simulink model "position_velocity_current_control"  (R2024b)
settings: Solver=VariableStepAuto  StartTime=0.0  StopTime=50  FixedStep=1e-5  RelTol=1e-3
values from neighbouring files (symbols this model uses):
  enable_saturators = true    [tuning.m]
  sinusoidal_trajectory = matlabFunction(sinusoidal_trajectory,Vars=[t, f, A])    [trajectories.m]
undefined symbols (not defined in the file or in its folder): b, J, K, Kv, V_nominal
libraries: fl_lib x22, cstblocks x16, nesl_utility x12, ee_lib x2
settings Model: Creator=frenci  LastModifiedBy=enrico
settings RTWCC: GPUComputeCapability=3.5

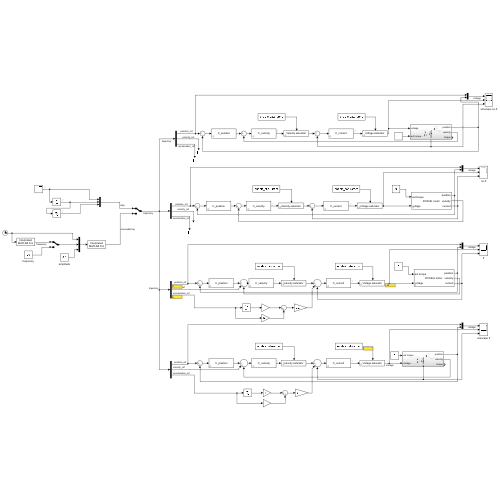
[thumbnail: Simulink's stored preview of the top-level diagram]
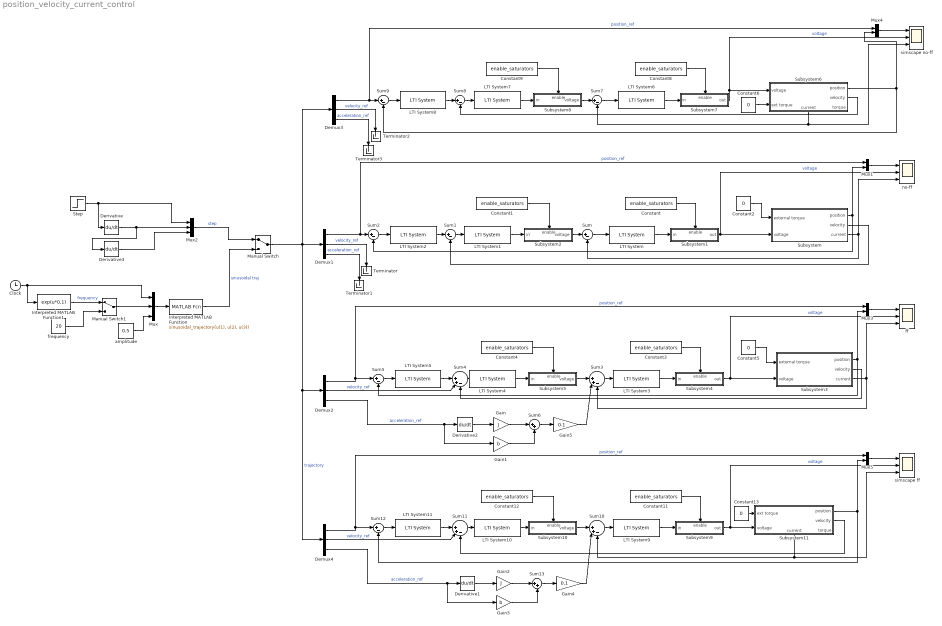
== system position_velocity_current_control ==
  Clock : Clock
  Constant{,1,3..4,8..9,11..12} (8 alike) : Constant  Value=enable_saturators
  Constant{2,5..6,13} (4 alike) : Constant  Value=0
  Demux{1..4} (4 alike) : Demux  Outputs=3
  Derivative : Derivative  CoefficientInTFapproximation=1000
  Derivative1 : Derivative
  Derivative2 : Derivative
  Derivative3 : Derivative  CoefficientInTFapproximation=1000
  Gain : Gain  Gain=J
  Gain1 : Gain  Gain=b
  Gain2 : Gain  Gain=J
  Gain3 : Gain  Gain=b
  Gain4 : Gain  Gain=0.1
  Gain5 : Gain  Gain=0.1
  Interpreted MATLAB Function : MATLABFcn  MATLABFcn=sinusoidal_trajectory(u(1), u(2), u(3))
  Interpreted MATLAB Function1 : MATLABFcn  MATLABFcn=exp(u*0.1)
  LTI System{,3,6,9} (4 alike) : cstblocks/LTI System  sys=C_current  IC=[]  PadeOrder=0
  LTI System{1,4,7,10} (4 alike) : cstblocks/LTI System  sys=C_velocity  IC=[]  PadeOrder=0
  LTI System{2,5,8,11} (4 alike) : cstblocks/LTI System  sys=C_position  IC=[]  PadeOrder=0
  Manual Switch : ManualSwitch
  Manual Switch1 : ManualSwitch
  Mux : Mux  Inputs=3
  Mux{1,3..5} (4 alike) : Mux  Inputs=2
  Mux2 : Mux  Inputs=3
  Step : Step  Time=0.5  SampleTime=0
  Subsystem : Subsystem
      mask Display:
      | disp('DCX22L motor');
      | 
      | port_label('output', 1, 'position');
      | port_label('output', 2, 'velocity');
      | port_label('output', 3, 'current');
      | 
      | port_label('input', 1, 'ext torque');
      | port_label('input', 2, 'voltage');
  Subsystem1 : Subsystem
      settings: PortSchema="{\"entries\":[{\"content\":{\"sides\":[{\"content\":{\"connectorIds\":[\"In1\"]},\"type\":\"ConnectorPlacement.EquallySpacedRectSide\",\"uuid\":\"5670bc23-5208-4592-a101-65e5ca02f12e\"},{\"content\":{\"connectorIds\":[\"Out1\"],\"side\":\"RIGHT\"},\"type\":\"ConnectorPlacement.EquallySpacedRectSide\",\"uuid\":\"ade26b55-5ce8-40ce-8bb9-a19330a12934\"},{\"content\":{\"connectorIds\":[\"In2\"],\"side\":\"TOP\"},\"type\":\"ConnectorPlacement.EquallySpacedRectSide\",\"uuid\":\"b961c51e-f004-41f7-8ef2-708d4a781ba3\"}]},\"type\":\"ConnectorPlacement.EquallySpacedConnector\",\"uuid\":\"606723ef-bc2b-476a-806f-27cbba92a2c4\"}],\"packageUris\":[\"http://schema.mathworks.com/mf0/Connector/R2020b\"],\"version\":\"1.0\"}"
      mask Display: disp('Voltage saturator')
  Subsystem10 : Subsystem
      settings: PortSchema="{\"entries\":[{\"content\":{\"sides\":[{\"content\":{\"connectorIds\":[\"In1\"]},\"type\":\"ConnectorPlacement.EquallySpacedRectSide\",\"uuid\":\"5670bc23-5208-4592-a101-65e5ca02f12e\"},{\"content\":{\"connectorIds\":[\"Out1\"],\"side\":\"RIGHT\"},\"type\":\"ConnectorPlacement.EquallySpacedRectSide\",\"uuid\":\"ade26b55-5ce8-40ce-8bb9-a19330a12934\"},{\"content\":{\"connectorIds\":[\"In2\"],\"side\":\"TOP\"},\"type\":\"ConnectorPlacement.EquallySpacedRectSide\",\"uuid\":\"b961c51e-f004-41f7-8ef2-708d4a781ba3\"}]},\"type\":\"ConnectorPlacement.EquallySpacedConnector\",\"uuid\":\"606723ef-bc2b-476a-806f-27cbba92a2c4\"}],\"packageUris\":[\"http://schema.mathworks.com/mf0/Connector/R2020b\"],\"version\":\"1.0\"}"
      mask Display: disp('Velocity saturator')
  Subsystem11 : Subsystem
      settings: PortSchema="{\"entries\":[{\"content\":{\"sides\":[{\"content\":{\"connectorIds\":[\"In1\",\"In2\"]},\"type\":\"ConnectorPlacement.EquallySpacedRectSide\",\"uuid\":\"c67ff89c-931e-4bc2-864c-883be475405e\"},{\"content\":{\"connectorIds\":[\"Out1\",\"Out2\",\"Out3\"],\"side\":\"RIGHT\"},\"type\":\"ConnectorPlacement.EquallySpacedRectSide\",\"uuid\":\"fb005381-2940-49c3-8bd1-e171080baf17\"},{\"content\":{\"side\":\"TOP\"},\"type\":\"ConnectorPlacement.EquallySpacedRectSide\",\"uuid\":\"7776594d-d5e0-4f5d-a5af-57046ad01644\"},{\"content\":{\"connectorIds\":[\"Out4\"],\"side\":\"BOTTOM\"},\"type\":\"ConnectorPlacement.EquallySpacedRectSide\",\"uuid\":\"24f18840-e2d9-4fce-8caf-60e308a91e4e\"}]},\"type\":\"ConnectorPlacement.EquallySpacedConnector\",\"uuid\":\"98be6553-19ec-40f8-9ca9-83476df98897\"}],\"packageUris\":[\"http://schema.mathworks.com/mf0/Connector/R2020b\"],\"version\":\"1.0\"}"
  Subsystem2 : Subsystem
      settings: PortSchema="{\"entries\":[{\"content\":{\"sides\":[{\"content\":{\"connectorIds\":[\"In1\"]},\"type\":\"ConnectorPlacement.EquallySpacedRectSide\",\"uuid\":\"5670bc23-5208-4592-a101-65e5ca02f12e\"},{\"content\":{\"connectorIds\":[\"Out1\"],\"side\":\"RIGHT\"},\"type\":\"ConnectorPlacement.EquallySpacedRectSide\",\"uuid\":\"ade26b55-5ce8-40ce-8bb9-a19330a12934\"},{\"content\":{\"connectorIds\":[\"In2\"],\"side\":\"TOP\"},\"type\":\"ConnectorPlacement.EquallySpacedRectSide\",\"uuid\":\"b961c51e-f004-41f7-8ef2-708d4a781ba3\"}]},\"type\":\"ConnectorPlacement.EquallySpacedConnector\",\"uuid\":\"606723ef-bc2b-476a-806f-27cbba92a2c4\"}],\"packageUris\":[\"http://schema.mathworks.com/mf0/Connector/R2020b\"],\"version\":\"1.0\"}"
      mask Display: disp('Velocity saturator')
  Subsystem3 : Subsystem
      mask Display:
      | disp('DCX22L motor');
      | 
      | port_label('output', 1, 'position');
      | port_label('output', 2, 'velocity');
      | port_label('output', 3, 'current');
      | 
      | port_label('input', 1, 'ext torque');
      | port_label('input', 2, 'voltage');
  Subsystem4 : Subsystem
      settings: PortSchema="{\"entries\":[{\"content\":{\"sides\":[{\"content\":{\"connectorIds\":[\"In1\"]},\"type\":\"ConnectorPlacement.EquallySpacedRectSide\",\"uuid\":\"5670bc23-5208-4592-a101-65e5ca02f12e\"},{\"content\":{\"connectorIds\":[\"Out1\"],\"side\":\"RIGHT\"},\"type\":\"ConnectorPlacement.EquallySpacedRectSide\",\"uuid\":\"ade26b55-5ce8-40ce-8bb9-a19330a12934\"},{\"content\":{\"connectorIds\":[\"In2\"],\"side\":\"TOP\"},\"type\":\"ConnectorPlacement.EquallySpacedRectSide\",\"uuid\":\"b961c51e-f004-41f7-8ef2-708d4a781ba3\"}]},\"type\":\"ConnectorPlacement.EquallySpacedConnector\",\"uuid\":\"606723ef-bc2b-476a-806f-27cbba92a2c4\"}],\"packageUris\":[\"http://schema.mathworks.com/mf0/Connector/R2020b\"],\"version\":\"1.0\"}"
      mask Display: disp('Voltage saturator')
  Subsystem5 : Subsystem
      settings: PortSchema="{\"entries\":[{\"content\":{\"sides\":[{\"content\":{\"connectorIds\":[\"In1\"]},\"type\":\"ConnectorPlacement.EquallySpacedRectSide\",\"uuid\":\"5670bc23-5208-4592-a101-65e5ca02f12e\"},{\"content\":{\"connectorIds\":[\"Out1\"],\"side\":\"RIGHT\"},\"type\":\"ConnectorPlacement.EquallySpacedRectSide\",\"uuid\":\"ade26b55-5ce8-40ce-8bb9-a19330a12934\"},{\"content\":{\"connectorIds\":[\"In2\"],\"side\":\"TOP\"},\"type\":\"ConnectorPlacement.EquallySpacedRectSide\",\"uuid\":\"b961c51e-f004-41f7-8ef2-708d4a781ba3\"}]},\"type\":\"ConnectorPlacement.EquallySpacedConnector\",\"uuid\":\"606723ef-bc2b-476a-806f-27cbba92a2c4\"}],\"packageUris\":[\"http://schema.mathworks.com/mf0/Connector/R2020b\"],\"version\":\"1.0\"}"
      mask Display: disp('Velocity saturator')
  Subsystem6 : Subsystem
      settings: PortSchema="{\"entries\":[{\"content\":{\"sides\":[{\"content\":{\"connectorIds\":[\"In1\",\"In2\"]},\"type\":\"ConnectorPlacement.EquallySpacedRectSide\",\"uuid\":\"c67ff89c-931e-4bc2-864c-883be475405e\"},{\"content\":{\"connectorIds\":[\"Out1\",\"Out2\",\"Out3\"],\"side\":\"RIGHT\"},\"type\":\"ConnectorPlacement.EquallySpacedRectSide\",\"uuid\":\"fb005381-2940-49c3-8bd1-e171080baf17\"},{\"content\":{\"side\":\"TOP\"},\"type\":\"ConnectorPlacement.EquallySpacedRectSide\",\"uuid\":\"7776594d-d5e0-4f5d-a5af-57046ad01644\"},{\"content\":{\"connectorIds\":[\"Out4\"],\"side\":\"BOTTOM\"},\"type\":\"ConnectorPlacement.EquallySpacedRectSide\",\"uuid\":\"24f18840-e2d9-4fce-8caf-60e308a91e4e\"}]},\"type\":\"ConnectorPlacement.EquallySpacedConnector\",\"uuid\":\"98be6553-19ec-40f8-9ca9-83476df98897\"}],\"packageUris\":[\"http://schema.mathworks.com/mf0/Connector/R2020b\"],\"version\":\"1.0\"}"
  Subsystem7 : Subsystem
      settings: PortSchema="{\"entries\":[{\"content\":{\"sides\":[{\"content\":{\"connectorIds\":[\"In1\"]},\"type\":\"ConnectorPlacement.EquallySpacedRectSide\",\"uuid\":\"5670bc23-5208-4592-a101-65e5ca02f12e\"},{\"content\":{\"connectorIds\":[\"Out1\"],\"side\":\"RIGHT\"},\"type\":\"ConnectorPlacement.EquallySpacedRectSide\",\"uuid\":\"ade26b55-5ce8-40ce-8bb9-a19330a12934\"},{\"content\":{\"connectorIds\":[\"In2\"],\"side\":\"TOP\"},\"type\":\"ConnectorPlacement.EquallySpacedRectSide\",\"uuid\":\"b961c51e-f004-41f7-8ef2-708d4a781ba3\"}]},\"type\":\"ConnectorPlacement.EquallySpacedConnector\",\"uuid\":\"606723ef-bc2b-476a-806f-27cbba92a2c4\"}],\"packageUris\":[\"http://schema.mathworks.com/mf0/Connector/R2020b\"],\"version\":\"1.0\"}"
      mask Display: disp('Voltage saturator')
  Subsystem8 : Subsystem
      settings: PortSchema="{\"entries\":[{\"content\":{\"sides\":[{\"content\":{\"connectorIds\":[\"In1\"]},\"type\":\"ConnectorPlacement.EquallySpacedRectSide\",\"uuid\":\"5670bc23-5208-4592-a101-65e5ca02f12e\"},{\"content\":{\"connectorIds\":[\"Out1\"],\"side\":\"RIGHT\"},\"type\":\"ConnectorPlacement.EquallySpacedRectSide\",\"uuid\":\"ade26b55-5ce8-40ce-8bb9-a19330a12934\"},{\"content\":{\"connectorIds\":[\"In2\"],\"side\":\"TOP\"},\"type\":\"ConnectorPlacement.EquallySpacedRectSide\",\"uuid\":\"b961c51e-f004-41f7-8ef2-708d4a781ba3\"}]},\"type\":\"ConnectorPlacement.EquallySpacedConnector\",\"uuid\":\"606723ef-bc2b-476a-806f-27cbba92a2c4\"}],\"packageUris\":[\"http://schema.mathworks.com/mf0/Connector/R2020b\"],\"version\":\"1.0\"}"
      mask Display: disp('Velocity saturator')
  Subsystem9 : Subsystem
      settings: PortSchema="{\"entries\":[{\"content\":{\"sides\":[{\"content\":{\"connectorIds\":[\"In1\"]},\"type\":\"ConnectorPlacement.EquallySpacedRectSide\",\"uuid\":\"5670bc23-5208-4592-a101-65e5ca02f12e\"},{\"content\":{\"connectorIds\":[\"Out1\"],\"side\":\"RIGHT\"},\"type\":\"ConnectorPlacement.EquallySpacedRectSide\",\"uuid\":\"ade26b55-5ce8-40ce-8bb9-a19330a12934\"},{\"content\":{\"connectorIds\":[\"In2\"],\"side\":\"TOP\"},\"type\":\"ConnectorPlacement.EquallySpacedRectSide\",\"uuid\":\"b961c51e-f004-41f7-8ef2-708d4a781ba3\"}]},\"type\":\"ConnectorPlacement.EquallySpacedConnector\",\"uuid\":\"606723ef-bc2b-476a-806f-27cbba92a2c4\"}],\"packageUris\":[\"http://schema.mathworks.com/mf0/Connector/R2020b\"],\"version\":\"1.0\"}"
      mask Display: disp('Voltage saturator')
  Sum{,1..2,5,7..9,12} (8 alike) : Sum  Inputs=|+-
  Sum{3..4,10..11} (4 alike) : Sum  Inputs=||++-
  Sum13 : Sum  Inputs=|++
  Sum6 : Sum  Inputs=|++
  Terminator{,1..3} (4 alike) : Terminator
  amplitude : Constant  Value=0.5
  ff : Scope  NumInputPorts=3
  frequency : Constant  Value=20
  no-ff : Scope  NumInputPorts=3
  simscape ff : Scope  NumInputPorts=3
  simscape no-ff : Scope  NumInputPorts=3
  wires:
  LTI System/1 -> Subsystem1/1(in)
  Subsystem1/1(out) -> no-ff/2, Subsystem/2(voltage)  "voltage"
  Sum/1 -> LTI System/1
  Subsystem/3(current) -> Sum/2, no-ff/3
  Sum1/1 -> LTI System1/1
  LTI System1/1 -> Subsystem2/1(in)
  Subsystem2/1(voltage) -> Sum/1
  LTI System2/1 -> Sum1/1
  Subsystem/2(velocity) -> Sum1/2
  Subsystem/1(position) -> Mux1/2, Sum2/2
  Sum2/1 -> LTI System2/1
  Demux1/1 -> Mux1/1, Sum2/1  "position_ref"
  Mux/1 -> Interpreted MATLAB Function/1
  Clock/1 -> Interpreted MATLAB Function1/1, Mux/1
  Manual Switch1/1 -> Mux/2
  Interpreted MATLAB Function/1 -> Manual Switch/2  "sinusoidal traj"
  amplitude/1 -> Mux/3
  Constant2/1 -> Subsystem/1(external torque)
  Constant/1 -> Subsystem1/2(enable)
  Constant1/1 -> Subsystem2/2(enable)
  Mux1/1 -> no-ff/1
  Step/1 -> Derivative/1, Mux2/1
  Mux2/1 -> Manual Switch/1  "step"
  Constant4/1 -> Subsystem5/2(enable)
  Constant5/1 -> Subsystem3/1(external torque)
  Subsystem3/3(current) -> ff/3, Sum3/3
  Constant3/1 -> Subsystem4/2(enable)
  Subsystem5/1(voltage) -> Sum3/1
  LTI System5/1 -> Sum4/1
  Demux2/1 -> Mux3/1, Sum5/1  "position_ref"
  Subsystem4/1(out) -> ff/2, Subsystem3/2(voltage)  "voltage"
  Subsystem3/1(position) -> Mux3/2, Sum5/2
  LTI System4/1 -> Subsystem5/1(in)
  LTI System3/1 -> Subsystem4/1(in)
  Sum3/1 -> LTI System3/1
  Sum4/1 -> LTI System4/1
  Subsystem3/2(velocity) -> Sum4/3
  Sum5/1 -> LTI System5/1
  Demux2/2 -> Sum4/2  "velocity_ref"
  Demux2/3 -> Derivative2/1, Gain1/1  "acceleration_ref"
  Derivative2/1 -> Gain/1
  Gain1/1 -> Sum6/2
  Gain/1 -> Sum6/1
  Sum6/1 -> Gain5/1
  Demux1/2 -> Terminator/1  "velocity_ref"
  Mux3/1 -> ff/1
  Demux1/3 -> Terminator1/1  "acceleration_ref"
  Subsystem6/4(current) -> simscape no-ff/3, Sum7/2
  Constant8/1 -> Subsystem7/2(enable)
  LTI System8/1 -> Sum8/1
  Mux4/1 -> simscape no-ff/1
  Subsystem8/1(voltage) -> Sum7/1
  Demux3/1 -> Mux4/1, Sum9/1  "position_ref"
  Demux3/2 -> Terminator2/1  "velocity_ref"
  Sum8/1 -> LTI System7/1
  Subsystem7/1(out) -> simscape no-ff/2, Subsystem6/1(voltage)  "voltage"
  Demux3/3 -> Terminator3/1  "acceleration_ref"
  LTI System6/1 -> Subsystem7/1(in)
  Constant9/1 -> Subsystem8/2(enable)
  LTI System7/1 -> Subsystem8/1(in)
  Sum7/1 -> LTI System6/1
  Sum9/1 -> LTI System8/1
  LTI System11/1 -> Sum11/1
  Constant12/1 -> Subsystem10/2(enable)
  Constant11/1 -> Subsystem9/2(enable)
  Sum12/1 -> LTI System11/1
  Subsystem11/2(velocity) -> Sum11/3
  Sum10/1 -> LTI System9/1
  LTI System9/1 -> Subsystem9/1(in)
  LTI System10/1 -> Subsystem10/1(in)
  Gain2/1 -> Sum13/1
  Subsystem9/1(out) -> Subsystem11/2(voltage), simscape ff/2  "voltage"
  Demux4/1 -> Mux5/1, Sum12/1  "position_ref"
  Subsystem10/1(voltage) -> Sum10/1
  Sum11/1 -> LTI System10/1
  Derivative1/1 -> Gain2/1
  Sum13/1 -> Gain4/1
  Mux5/1 -> simscape ff/1
  Demux4/2 -> Sum11/2  "velocity_ref"
  Subsystem11/1(position) -> Sum12/2, Mux5/2
  Gain3/1 -> Sum13/2
  Manual Switch/1 -> Demux3/1, Demux4/1, Demux2/1, Demux1/1  "trajectory"
  Subsystem11/4(current) -> simscape ff/3, Sum10/3
  Demux4/3 -> Derivative1/1, Gain3/1  "acceleration_ref"
  Derivative/1 -> Derivative3/1, Mux2/2
  Derivative3/1 -> Mux2/3
  Subsystem6/2(velocity) -> Sum8/2
  Subsystem6/1(position) -> Sum9/2, Mux4/2
  Constant6/1 -> Subsystem6/2(ext torque)
  Constant13/1 -> Subsystem11/1(ext torque)
  Gain4/1 -> Sum10/2
  Interpreted MATLAB Function1/1 -> Manual Switch1/1  "frequency"
  frequency/1 -> Manual Switch1/2
  Gain5/1 -> Sum3/2

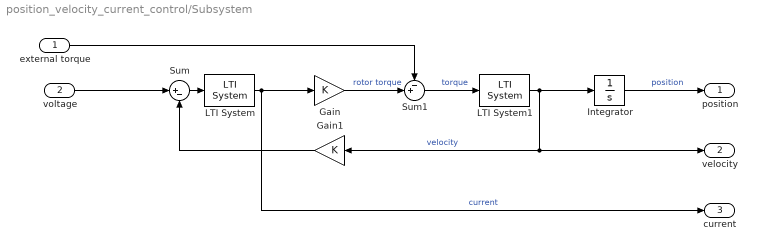
== system position_velocity_current_control/Subsystem ==
  external torque : Inport
  voltage : Inport  Port=2
  Gain : Gain  Gain=K
  Gain1 : Gain  Gain=K
  Integrator : Integrator
  LTI System : cstblocks/LTI System  sys=El  IC=[]  PadeOrder=0
  LTI System1 : cstblocks/LTI System  sys=Me  IC=[]  PadeOrder=0
  Sum : Sum  Inputs=|+-
  Sum1 : Sum  Inputs=-+|
  position : Outport
  velocity : Outport  Port=2
  current : Outport  Port=3
  wires:
  LTI System/1 -> current/1, Gain/1  "current"
  Gain1/1 -> Sum/2
  Integrator/1 -> position/1  "position"
  voltage/1 -> Sum/1
  Gain/1 -> Sum1/2  "rotor torque"
  Sum1/1 -> LTI System1/1  "torque"
  Sum/1 -> LTI System/1
  LTI System1/1 -> velocity/1, Gain1/1, Integrator/1  "velocity"
  external torque/1 -> Sum1/1

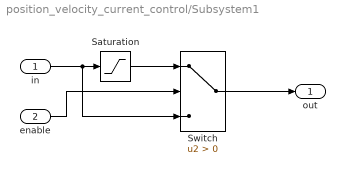
== system position_velocity_current_control/Subsystem1 ==
  in : Inport
  enable : Inport  Port=2
  Saturation : Saturate  UpperLimit=V_nominal  LowerLimit=-V_nominal
  Switch : Switch  Criteria=u2 > Threshold  SaturateOnIntegerOverflow=off  InputSameDT=off
  out : Outport
  wires:
  in/1 -> Switch/3, Saturation/1
  enable/1 -> Switch/2
  Switch/1 -> out/1
  Saturation/1 -> Switch/1

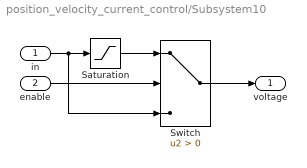
== system position_velocity_current_control/Subsystem10 ==
  in : Inport
  enable : Inport  Port=2
  Saturation : Saturate  UpperLimit=V_nominal*Kv*0.10472  LowerLimit=-V_nominal*Kv*0.10472
  Switch : Switch  Criteria=u2 > Threshold  SaturateOnIntegerOverflow=off  InputSameDT=off
  voltage : Outport
  wires:
  in/1 -> Switch/3, Saturation/1
  Switch/1 -> voltage/1
  Saturation/1 -> Switch/1
  enable/1 -> Switch/2

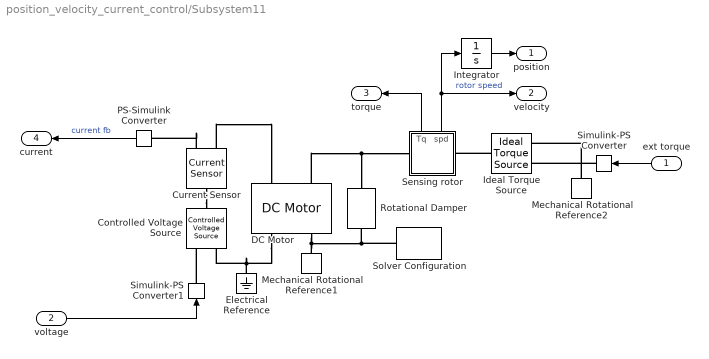
== system position_velocity_current_control/Subsystem11 ==
  ext torque : Inport
  voltage : Inport  Port=2
  Controlled Voltage Source : fl_lib/Electrical/Electrical Sources/Controlled Voltage Source
  Current Sensor : fl_lib/Electrical/Electrical Sensors/Current Sensor
  DC Motor : ee_lib/Electromechanical/Brushed Motors/DC Motor  field_option=ee.enum.field_option.pm  Rf=100 Ohm  Lf=1 H  Laf=0.15 H  If0=0 A  parameterization=ee.enum.dcparam_option.circuit_param  Ra=R Ohm  La=L H  emf_or_torque=ee.enum.emf_or_torque.kv  Kv=1/Kv V/rpm  Ki=6.876e-4 N*m/A  T_stall=0.24e-3 N*m  w_max=19100 rpm  w_rated=15000 rpm  P_rated=0.08 W  V_rated=1.5 V  lam_param=ee.enum.lam_param.current  i_noload="54.6  mA"  V_i_noload=18 V  J=J cm^2*g  lam=0 N*m*s/rad  speed0=0 rpm  t_fault_armature=1 s  t_fault_field=1 s  fault_action=simscape.enum.assert.action.none  alpha=3.93e-3 1/K  Tmeas=25 degC  thermal_mass=100 J/K  initial_temperature=25 degC
  Electrical Reference : fl_lib/Electrical/Electrical Elements/Electrical Reference
  Ideal Torque Source : fl_lib/Mechanical/Mechanical Sources/Ideal Torque Source
  Integrator : Integrator
  Mechanical Rotational Reference1 : fl_lib/Mechanical/Rotational Elements/Mechanical Rotational Reference
  Mechanical Rotational Reference2 : fl_lib/Mechanical/Rotational Elements/Mechanical Rotational Reference
  PS-Simulink Converter : nesl_utility/PS-Simulink Converter  PhysicalDomain=network_engine_domain  SubClassName=ps_output  LeftPortType=input  RightPortType=output  PseudoPeriodic=off  Frequencies=[]  VectorFormat=inherit  Unit=inherit  AffineConversion=off
  Rotational Damper : fl_lib/Mechanical/Rotational Elements/Rotational Damper  D=b N*m*s/rad  w_specify=off  w_priority=None  w=0 rad/s  w_nominal_specify=off  w_nominal_value=1  w_nominal_unit=rad/s  t_specify=off  t_priority=None  t=0 N*m  t_nominal_specify=off  t_nominal_value=1  t_nominal_unit=N*m
  Sensing rotor : Subsystem
      settings: PortSchema="{\"entries\":[{\"content\":{\"sides\":[{\"content\":{\"connectorIds\":[\"LConn1\"]},\"type\":\"ConnectorPlacement.EquallySpacedRectSide\",\"uuid\":\"9165a8ad-3db0-41c0-ab54-3b61ce0d4991\"},{\"content\":{\"connectorIds\":[\"RConn1\"],\"side\":\"RIGHT\"},\"type\":\"ConnectorPlacement.EquallySpacedRectSide\",\"uuid\":\"77dd0fe0-a538-4e9a-a5e5-b4e8faf0921d\"},{\"content\":{\"connectorIds\":[\"Out1\",\"Out2\"],\"side\":\"TOP\"},\"type\":\"ConnectorPlacement.EquallySpacedRectSide\",\"uuid\":\"6454db15-9e49-4f4a-bb19-0d462346e2ce\"},{\"content\":{\"connectorIds\":[],\"side\":\"BOTTOM\"},\"type\":\"ConnectorPlacement.EquallySpacedRectSide\",\"uuid\":\"205718cf-2aa2-41bb-bfb4-a63575d19392\"}]},\"type\":\"ConnectorPlacement.EquallySpacedConnector\",\"uuid\":\"b0e56a53-c948-4e6a-adfb-62f2ad9887fa\"}],\"packageUris\":[\"http://schema.mathworks.com/mf0/Connector/R2020b\"],\"version\":\"1.0\"}"
  Simulink-PS Converter : nesl_utility/Simulink-PS Converter  PhysicalDomain=network_engine_domain  SubClassName=ps_input  LeftPortType=input  RightPortType=output  PseudoPeriodic=off  Frequencies=[]  NoiseDistribution=none  NoiseParameters=[]  Unit=1  AffineConversion=off  FilteringAndDerivatives=provide  SimscapeFilterOrder=1  InputFilterTimeConstant=0.001  UdotUserProvided=0
  Simulink-PS Converter1 : nesl_utility/Simulink-PS Converter  PhysicalDomain=network_engine_domain  SubClassName=ps_input  LeftPortType=input  RightPortType=output  PseudoPeriodic=off  Frequencies=[]  NoiseDistribution=none  NoiseParameters=[]  Unit=1  AffineConversion=off  FilteringAndDerivatives=zero  SimscapeFilterOrder=1  InputFilterTimeConstant=0.001  UdotUserProvided=0
  Solver Configuration : nesl_utility/Solver Configuration  PhysicalDomain=network_engine_domain  SubClassName=solver  LeftPortType=input  RightPortType=generic  Tones=[]  Harmonics=[]  SimulateNoise=off  Profile=off  UseLocalSampling=off  EnableSwitchedLinearOptims=on  FrequencyDomain=off  UseCCode=off  RelTol=0.001  AbsTol=0.001  MinStep=1e-09  ToWorkspace=off  RevertToSquareIcSolve=off  NumHomotopyIterations=100  PhasorMode=off  PhasorModeNumHarmonics=1  ConsistencySolver=NEWTON_XTOL_AFTER_FTOL  IndexReductionMethod=DerivativeReplacement  DoDC=off  ResidualTolerance=1e-09  ConsistencyTolSource=GLOBAL  ConsistencyAbsTol=0.001  ConsistencyRelTol=0.001  ConsistencyTolFactor=0.000001  UseLocalSolver=off  LocalSolverChoice=NE_BACKWARD_EULER_ADVANCER  ResolveIndetEquations=on  FunctionEvalNumThread=1  LocalSolverSampleTime=0.001  DoFixedCost=off  MaxNonlinIter=3  MaxModeIter=2  ComputeImpulses=off  ImpulseIterations=2  LinearAlgebra=auto  LinearAlgebraNumThread=0  EquationFormulation=NE_TIME_EF  DelaysMemoryBudget=1024  AutomaticFiltering=on  FilteringTimeConstant=0.001  PartitionStorageMethod=AS_NEEDED  PartitionMemoryBudget=1024  PartitionMethod=ROBUST  MultibodyUseLocalSolver=off  MultibodyLocalSolverChoice=ODE1  MultibodyLocalSolverSampleTime=0.001
  position : Outport
  velocity : Outport  Port=2
  torque : Outport  Port=3
  current : Outport  Port=4
  wires:
  Sensing rotor/1(Tq) -> torque/1
  PS-Simulink Converter/1 -> current/1  "current fb"
  Sensing rotor/2(spd) -> Integrator/1, velocity/1  "rotor speed"
  voltage/1 -> Simulink-PS Converter1/1
  ext torque/1 -> Simulink-PS Converter/1
  Integrator/1 -> position/1
  connections:
  DC Motor/RConn1 -- Electrical Reference/LConn1 -- Controlled Voltage Source/RConn2
  Current Sensor/RConn1 -- PS-Simulink Converter/LConn1
  Simulink-PS Converter1/RConn1 -- Controlled Voltage Source/RConn1
  DC Motor/LConn2 -- Rotational Damper/LConn1 -- Sensing rotor/LConn1
  DC Motor/RConn2 -- Mechanical Rotational Reference1/LConn1 -- Solver Configuration/RConn1 -- Rotational Damper/RConn1
  Current Sensor/RConn2 -- DC Motor/LConn1
  Ideal Torque Source/LConn1 -- Sensing rotor/RConn1
  Current Sensor/LConn1 -- Controlled Voltage Source/LConn1
  Simulink-PS Converter/RConn1 -- Ideal Torque Source/RConn1
  Mechanical Rotational Reference2/LConn1 -- Ideal Torque Source/RConn2

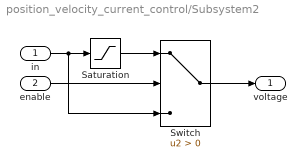
== system position_velocity_current_control/Subsystem2 ==
  in : Inport
  enable : Inport  Port=2
  Saturation : Saturate  UpperLimit=V_nominal*Kv*0.10472  LowerLimit=-V_nominal*Kv*0.10472
  Switch : Switch  Criteria=u2 > Threshold  SaturateOnIntegerOverflow=off  InputSameDT=off
  voltage : Outport
  wires:
  in/1 -> Switch/3, Saturation/1
  Switch/1 -> voltage/1
  Saturation/1 -> Switch/1
  enable/1 -> Switch/2

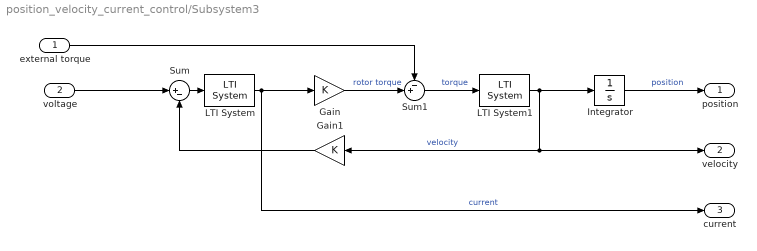
== system position_velocity_current_control/Subsystem3 ==
  external torque : Inport
  voltage : Inport  Port=2
  Gain : Gain  Gain=K
  Gain1 : Gain  Gain=K
  Integrator : Integrator
  LTI System : cstblocks/LTI System  sys=El  IC=[]  PadeOrder=0
  LTI System1 : cstblocks/LTI System  sys=Me  IC=[]  PadeOrder=0
  Sum : Sum  Inputs=|+-
  Sum1 : Sum  Inputs=-+|
  position : Outport
  velocity : Outport  Port=2
  current : Outport  Port=3
  wires:
  LTI System/1 -> current/1, Gain/1  "current"
  Gain1/1 -> Sum/2
  Integrator/1 -> position/1  "position"
  voltage/1 -> Sum/1
  Gain/1 -> Sum1/2  "rotor torque"
  Sum1/1 -> LTI System1/1  "torque"
  Sum/1 -> LTI System/1
  LTI System1/1 -> velocity/1, Gain1/1, Integrator/1  "velocity"
  external torque/1 -> Sum1/1

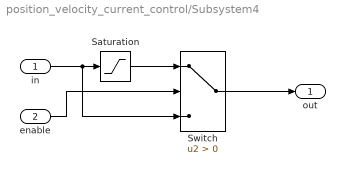
== system position_velocity_current_control/Subsystem4 ==
  in : Inport
  enable : Inport  Port=2
  Saturation : Saturate  UpperLimit=V_nominal  LowerLimit=-V_nominal  ZeroCross=off
  Switch : Switch  Criteria=u2 > Threshold  SaturateOnIntegerOverflow=off  InputSameDT=off
  out : Outport
  wires:
  in/1 -> Switch/3, Saturation/1
  enable/1 -> Switch/2
  Switch/1 -> out/1
  Saturation/1 -> Switch/1

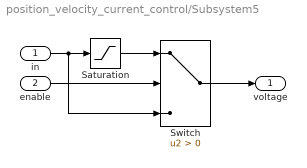
== system position_velocity_current_control/Subsystem5 ==
  in : Inport
  enable : Inport  Port=2
  Saturation : Saturate  UpperLimit=V_nominal*Kv*0.10472  LowerLimit=-V_nominal*Kv*0.10472
  Switch : Switch  Criteria=u2 > Threshold  SaturateOnIntegerOverflow=off  InputSameDT=off
  voltage : Outport
  wires:
  in/1 -> Switch/3, Saturation/1
  Switch/1 -> voltage/1
  Saturation/1 -> Switch/1
  enable/1 -> Switch/2

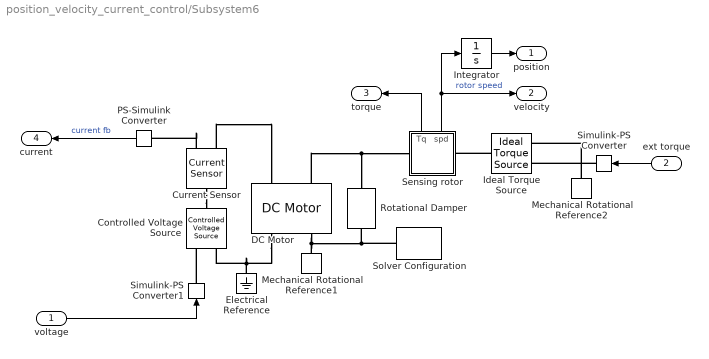
== system position_velocity_current_control/Subsystem6 ==
  voltage : Inport
  ext torque : Inport  Port=2
  Controlled Voltage Source : fl_lib/Electrical/Electrical Sources/Controlled Voltage Source
  Current Sensor : fl_lib/Electrical/Electrical Sensors/Current Sensor
  DC Motor : ee_lib/Electromechanical/Brushed Motors/DC Motor  field_option=ee.enum.field_option.pm  Rf=100 Ohm  Lf=1 H  Laf=0.15 H  If0=0 A  parameterization=ee.enum.dcparam_option.circuit_param  Ra=R Ohm  La=L H  emf_or_torque=ee.enum.emf_or_torque.kv  Kv=1/Kv V/rpm  Ki=6.876e-4 N*m/A  T_stall=0.24e-3 N*m  w_max=19100 rpm  w_rated=15000 rpm  P_rated=0.08 W  V_rated=1.5 V  lam_param=ee.enum.lam_param.current  i_noload="54.6  mA"  V_i_noload=18 V  J=J cm^2*g  lam=0 N*m*s/rad  speed0=0 rpm  t_fault_armature=1 s  t_fault_field=1 s  fault_action=simscape.enum.assert.action.none  alpha=3.93e-3 1/K  Tmeas=25 degC  thermal_mass=100 J/K  initial_temperature=25 degC
  Electrical Reference : fl_lib/Electrical/Electrical Elements/Electrical Reference
  Ideal Torque Source : fl_lib/Mechanical/Mechanical Sources/Ideal Torque Source
  Integrator : Integrator
  Mechanical Rotational Reference1 : fl_lib/Mechanical/Rotational Elements/Mechanical Rotational Reference
  Mechanical Rotational Reference2 : fl_lib/Mechanical/Rotational Elements/Mechanical Rotational Reference
  PS-Simulink Converter : nesl_utility/PS-Simulink Converter  PhysicalDomain=network_engine_domain  SubClassName=ps_output  LeftPortType=input  RightPortType=output  PseudoPeriodic=off  Frequencies=[]  VectorFormat=inherit  Unit=inherit  AffineConversion=off
  Rotational Damper : fl_lib/Mechanical/Rotational Elements/Rotational Damper  D=b N*m*s/rad  w_specify=off  w_priority=None  w=0 rad/s  w_nominal_specify=off  w_nominal_value=1  w_nominal_unit=rad/s  t_specify=off  t_priority=None  t=0 N*m  t_nominal_specify=off  t_nominal_value=1  t_nominal_unit=N*m
  Sensing rotor : Subsystem
      settings: PortSchema="{\"entries\":[{\"content\":{\"sides\":[{\"content\":{\"connectorIds\":[\"LConn1\"]},\"type\":\"ConnectorPlacement.EquallySpacedRectSide\",\"uuid\":\"9165a8ad-3db0-41c0-ab54-3b61ce0d4991\"},{\"content\":{\"connectorIds\":[\"RConn1\"],\"side\":\"RIGHT\"},\"type\":\"ConnectorPlacement.EquallySpacedRectSide\",\"uuid\":\"77dd0fe0-a538-4e9a-a5e5-b4e8faf0921d\"},{\"content\":{\"connectorIds\":[\"Out1\",\"Out2\"],\"side\":\"TOP\"},\"type\":\"ConnectorPlacement.EquallySpacedRectSide\",\"uuid\":\"6454db15-9e49-4f4a-bb19-0d462346e2ce\"},{\"content\":{\"connectorIds\":[],\"side\":\"BOTTOM\"},\"type\":\"ConnectorPlacement.EquallySpacedRectSide\",\"uuid\":\"205718cf-2aa2-41bb-bfb4-a63575d19392\"}]},\"type\":\"ConnectorPlacement.EquallySpacedConnector\",\"uuid\":\"b0e56a53-c948-4e6a-adfb-62f2ad9887fa\"}],\"packageUris\":[\"http://schema.mathworks.com/mf0/Connector/R2020b\"],\"version\":\"1.0\"}"
  Simulink-PS Converter : nesl_utility/Simulink-PS Converter  PhysicalDomain=network_engine_domain  SubClassName=ps_input  LeftPortType=input  RightPortType=output  PseudoPeriodic=off  Frequencies=[]  NoiseDistribution=none  NoiseParameters=[]  Unit=1  AffineConversion=off  FilteringAndDerivatives=provide  SimscapeFilterOrder=1  InputFilterTimeConstant=0.001  UdotUserProvided=0
  Simulink-PS Converter1 : nesl_utility/Simulink-PS Converter  PhysicalDomain=network_engine_domain  SubClassName=ps_input  LeftPortType=input  RightPortType=output  PseudoPeriodic=off  Frequencies=[]  NoiseDistribution=none  NoiseParameters=[]  Unit=1  AffineConversion=off  FilteringAndDerivatives=zero  SimscapeFilterOrder=1  InputFilterTimeConstant=0.001  UdotUserProvided=0
  Solver Configuration : nesl_utility/Solver Configuration  PhysicalDomain=network_engine_domain  SubClassName=solver  LeftPortType=input  RightPortType=generic  Tones=[]  Harmonics=[]  SimulateNoise=off  Profile=off  UseLocalSampling=off  EnableSwitchedLinearOptims=on  FrequencyDomain=off  UseCCode=off  RelTol=0.001  AbsTol=0.001  MinStep=1e-09  ToWorkspace=off  RevertToSquareIcSolve=off  NumHomotopyIterations=100  PhasorMode=off  PhasorModeNumHarmonics=1  ConsistencySolver=NEWTON_XTOL_AFTER_FTOL  IndexReductionMethod=DerivativeReplacement  DoDC=off  ResidualTolerance=1e-09  ConsistencyTolSource=GLOBAL  ConsistencyAbsTol=0.001  ConsistencyRelTol=0.001  ConsistencyTolFactor=0.000001  UseLocalSolver=off  LocalSolverChoice=NE_BACKWARD_EULER_ADVANCER  ResolveIndetEquations=on  FunctionEvalNumThread=1  LocalSolverSampleTime=0.001  DoFixedCost=off  MaxNonlinIter=3  MaxModeIter=2  ComputeImpulses=off  ImpulseIterations=2  LinearAlgebra=auto  LinearAlgebraNumThread=0  EquationFormulation=NE_TIME_EF  DelaysMemoryBudget=1024  AutomaticFiltering=on  FilteringTimeConstant=0.001  PartitionStorageMethod=AS_NEEDED  PartitionMemoryBudget=1024  PartitionMethod=ROBUST  MultibodyUseLocalSolver=off  MultibodyLocalSolverChoice=ODE1  MultibodyLocalSolverSampleTime=0.001
  position : Outport
  velocity : Outport  Port=2
  torque : Outport  Port=3
  current : Outport  Port=4
  wires:
  Sensing rotor/1(Tq) -> torque/1
  PS-Simulink Converter/1 -> current/1  "current fb"
  Sensing rotor/2(spd) -> Integrator/1, velocity/1  "rotor speed"
  voltage/1 -> Simulink-PS Converter1/1
  ext torque/1 -> Simulink-PS Converter/1
  Integrator/1 -> position/1
  connections:
  DC Motor/RConn1 -- Electrical Reference/LConn1 -- Controlled Voltage Source/RConn2
  Current Sensor/RConn1 -- PS-Simulink Converter/LConn1
  Simulink-PS Converter1/RConn1 -- Controlled Voltage Source/RConn1
  DC Motor/LConn2 -- Sensing rotor/LConn1 -- Rotational Damper/LConn1
  DC Motor/RConn2 -- Mechanical Rotational Reference1/LConn1 -- Solver Configuration/RConn1 -- Rotational Damper/RConn1
  Current Sensor/RConn2 -- DC Motor/LConn1
  Ideal Torque Source/LConn1 -- Sensing rotor/RConn1
  Current Sensor/LConn1 -- Controlled Voltage Source/LConn1
  Simulink-PS Converter/RConn1 -- Ideal Torque Source/RConn1
  Mechanical Rotational Reference2/LConn1 -- Ideal Torque Source/RConn2

== system position_velocity_current_control/Subsystem7 ==
  in : Inport
  enable : Inport  Port=2
  Saturation : Saturate  UpperLimit=V_nominal  LowerLimit=-V_nominal
  Switch : Switch  Criteria=u2 > Threshold  SaturateOnIntegerOverflow=off  InputSameDT=off
  out : Outport
  wires:
  in/1 -> Switch/3, Saturation/1
  enable/1 -> Switch/2
  Switch/1 -> out/1
  Saturation/1 -> Switch/1

== system position_velocity_current_control/Subsystem8 ==
  in : Inport
  enable : Inport  Port=2
  Saturation : Saturate  UpperLimit=V_nominal*Kv*0.10472  LowerLimit=-V_nominal*Kv*0.10472
  Switch : Switch  Criteria=u2 > Threshold  SaturateOnIntegerOverflow=off  InputSameDT=off
  voltage : Outport
  wires:
  in/1 -> Switch/3, Saturation/1
  Switch/1 -> voltage/1
  Saturation/1 -> Switch/1
  enable/1 -> Switch/2

== system position_velocity_current_control/Subsystem9 ==
  in : Inport
  enable : Inport  Port=2
  Saturation : Saturate  UpperLimit=V_nominal  LowerLimit=-V_nominal  ZeroCross=off
  Switch : Switch  Criteria=u2 > Threshold  SaturateOnIntegerOverflow=off  InputSameDT=off
  out : Outport
  wires:
  in/1 -> Switch/3, Saturation/1
  enable/1 -> Switch/2
  Switch/1 -> out/1
  Saturation/1 -> Switch/1

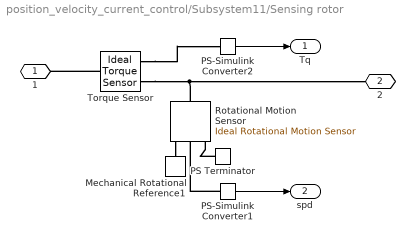
== system position_velocity_current_control/Subsystem11/Sensing rotor ==
  Mechanical Rotational Reference1 : fl_lib/Mechanical/Rotational Elements/Mechanical Rotational Reference
  PS Terminator : fl_lib/Physical Signals/Sinks/PS Terminator
  PS-Simulink Converter1 : nesl_utility/PS-Simulink Converter  PhysicalDomain=network_engine_domain  SubClassName=ps_output  LeftPortType=input  RightPortType=output  PseudoPeriodic=off  Frequencies=[]  VectorFormat=1-D array  Unit=rpm  AffineConversion=off
  PS-Simulink Converter2 : nesl_utility/PS-Simulink Converter  PhysicalDomain=network_engine_domain  SubClassName=ps_output  LeftPortType=input  RightPortType=output  PseudoPeriodic=off  Frequencies=[]  VectorFormat=1-D array  Unit=N*m  AffineConversion=off
  Rotational Motion Sensor : fl_lib/Mechanical/Mechanical Sensors/Ideal Rotational Motion Sensor  reference=foundation.enum.MeasurementReference.difference  acceleration_port=false  velocity_port=true  position_port=true  wrap_angle=simscape.enum.onoff.off  offset=0 rad
  Torque Sensor : fl_lib/Mechanical/Mechanical Sensors/Ideal Torque Sensor
  1 : PMIOPort  Side=Left
  2 : PMIOPort  Port=2  Side=Right
  Tq : Outport
  spd : Outport  Port=2
  wires:
  PS-Simulink Converter2/1 -> Tq/1
  PS-Simulink Converter1/1 -> spd/1
  connections:
  Rotational Motion Sensor/RConn1 -- Mechanical Rotational Reference1/LConn1
  Torque Sensor/LConn1 -- 1/RConn1
  Torque Sensor/RConn2 -- PS-Simulink Converter2/LConn1
  Rotational Motion Sensor/LConn1 -- 2/RConn1 -- Torque Sensor/RConn1
  PS-Simulink Converter1/LConn1 -- Rotational Motion Sensor/RConn2
  PS Terminator/LConn1 -- Rotational Motion Sensor/RConn3

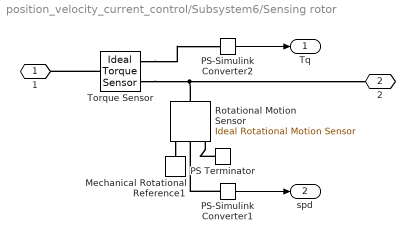
== system position_velocity_current_control/Subsystem6/Sensing rotor ==
  Mechanical Rotational Reference1 : fl_lib/Mechanical/Rotational Elements/Mechanical Rotational Reference
  PS Terminator : fl_lib/Physical Signals/Sinks/PS Terminator
  PS-Simulink Converter1 : nesl_utility/PS-Simulink Converter  PhysicalDomain=network_engine_domain  SubClassName=ps_output  LeftPortType=input  RightPortType=output  PseudoPeriodic=off  Frequencies=[]  VectorFormat=1-D array  Unit=rpm  AffineConversion=off
  PS-Simulink Converter2 : nesl_utility/PS-Simulink Converter  PhysicalDomain=network_engine_domain  SubClassName=ps_output  LeftPortType=input  RightPortType=output  PseudoPeriodic=off  Frequencies=[]  VectorFormat=1-D array  Unit=N*m  AffineConversion=off
  Rotational Motion Sensor : fl_lib/Mechanical/Mechanical Sensors/Ideal Rotational Motion Sensor  reference=foundation.enum.MeasurementReference.difference  acceleration_port=false  velocity_port=true  position_port=true  wrap_angle=simscape.enum.onoff.off  offset=0 rad
  Torque Sensor : fl_lib/Mechanical/Mechanical Sensors/Ideal Torque Sensor
  1 : PMIOPort  Side=Left
  2 : PMIOPort  Port=2  Side=Right
  Tq : Outport
  spd : Outport  Port=2
  wires:
  PS-Simulink Converter2/1 -> Tq/1
  PS-Simulink Converter1/1 -> spd/1
  connections:
  Rotational Motion Sensor/RConn1 -- Mechanical Rotational Reference1/LConn1
  Torque Sensor/LConn1 -- 1/RConn1
  Torque Sensor/RConn2 -- PS-Simulink Converter2/LConn1
  Rotational Motion Sensor/LConn1 -- 2/RConn1 -- Torque Sensor/RConn1
  PS-Simulink Converter1/LConn1 -- Rotational Motion Sensor/RConn2
  PS Terminator/LConn1 -- Rotational Motion Sensor/RConn3
